simulink model "model"  (R2023b)
settings: Solver=ode23tb  StartTime=0.0  StopTime=Tmdl  MaxStep=1e-3  RelTol=1e-3
undefined symbols (not defined in the file or in its folder): den, k, num
settings Model: Creator=deniskirbaba  LastModifiedBy=deniskirbaba

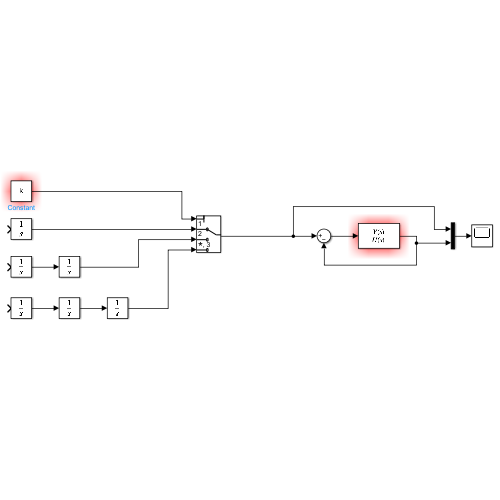
[thumbnail: Simulink's stored preview of the top-level diagram]
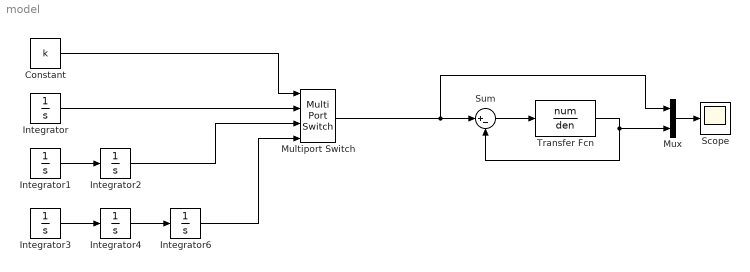
== system model ==
  Constant : Constant  Value=k
  Integrator : Integrator  InitialCondition=1
  Integrator1 : Integrator  InitialCondition=1
  Integrator2 : Integrator
  Integrator3 : Integrator  InitialCondition=1
  Integrator4 : Integrator
  Integrator6 : Integrator
  Multiport Switch : MultiPortSwitch  SaturateOnIntegerOverflow=off  InputSameDT=off
  Mux : Mux  Inputs=2
  Scope : Scope
  Sum : Sum  Inputs=|+-
  Transfer Fcn : TransferFcn  Numerator=num  Denominator=den
  wires:
  Sum/1 -> Transfer Fcn/1
  Transfer Fcn/1 -> Mux/2, Sum/2
  Mux/1 -> Scope/1
  Multiport Switch/1 -> Mux/1, Sum/1
  Integrator1/1 -> Integrator2/1
  Integrator3/1 -> Integrator4/1
  Integrator4/1 -> Integrator6/1
  Integrator/1 -> Multiport Switch/2
  Integrator2/1 -> Multiport Switch/3
  Integrator6/1 -> Multiport Switch/4
  Constant/1 -> Multiport Switch/1
